simulink library "flowColumnSpec_ul"  (R2022a)
settings: Solver=VariableStepAuto  StartTime=0.0  StopTime=10.0  RelTol=1e-3
undefined symbols (not defined in the file): env, flow, height
settings Model: Creator=M.Cobb  LastModifiedBy=adabney
settings SolverCC: AlgebraicLoopSolver=TrustRegion
settings DebuggingCC: UnconnectedInputMsg=warning  UnconnectedOutputMsg=warning  UnconnectedLineMsg=warning  SFMachineParentedDataDiag=warning  ArithmeticOperatorsInVariantConditions=warning
settings SFSimCC: CustomCodeUndefinedFunction=UseInterfaceOnly

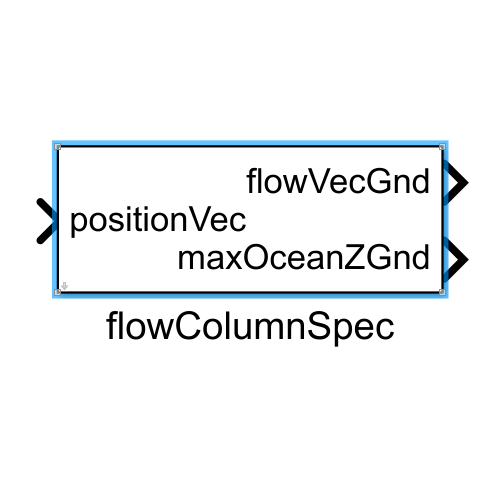
[thumbnail: Simulink's stored preview of the top-level diagram]
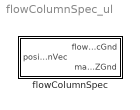
== system flowColumnSpec_ul ==
  flowColumnSpec : Subsystem  VariantControl=VSS_flowCalculation_constXYZT  mask{baseFlow=env.water}
      mask prompts: baseFlow "Base Flow"

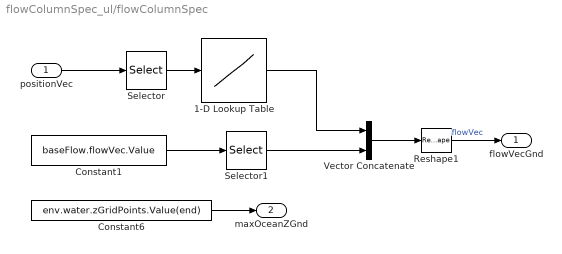
== system flowColumnSpec_ul/flowColumnSpec ==
  positionVec : Inport  PortDimensions=[3 1]
  1-D Lookup Table : Lookup_n-D  NumberOfTableDimensions=1  BreakpointsForDimension1=height  Table=flow  InternalRulePriority=Speed  RndMeth=Simplest
  Constant1 : Constant  Value=baseFlow.flowVec.Value
  Constant6 : Constant  Value=env.water.zGridPoints.Value(end)
  Reshape1 : Reshape  OutputDimensionality=Column vector (2-D)
  Selector : Selector  InputPortWidth=3  IndexOptions=Index vector (dialog)  Indices=3  OutputSizes=1
  Selector1 : Selector  InputPortWidth=3  IndexOptions=Index vector (dialog)  Indices=[2 3]  OutputSizes=1
  Vector Concatenate : Concatenate
  flowVecGnd : Outport  VectorParamsAs1DForOutWhenUnconnected=off
  maxOceanZGnd : Outport  Port=2  VectorParamsAs1DForOutWhenUnconnected=off
  wires:
  1-D Lookup Table/1 -> Vector Concatenate/1
  Constant1/1 -> Selector1/1
  Constant6/1 -> maxOceanZGnd/1
  Reshape1/1 -> flowVecGnd/1  "flowVec"
  positionVec/1 -> Selector/1
  Selector/1 -> 1-D Lookup Table/1
  Selector1/1 -> Vector Concatenate/2
  Vector Concatenate/1 -> Reshape1/1
